simulink model "Simplus_Dual_Automated"  (R2022b)
settings: Solver=ode3  StartTime=0.0  StopTime=35  FixedStep=Ts  RelTol=1e-3  EnableMultiTasking=on
InitFcn:
  | Ts = 100e-6;
model workspace (MAT data in the model file):
  Fbase = 50
  Filter_Ind = 0.00435
  Shunt_C = 2.2e-06
  Test_Interval = 5
  Ts = 0.0001
  VDCref = 48
undefined symbols (not defined in the file): DiscIntNeverNeededParam
libraries: rtpi x45, spsabctodq0Lib x4, spsdq0toabcLib x2, simulink x1
(part 2 of 2)

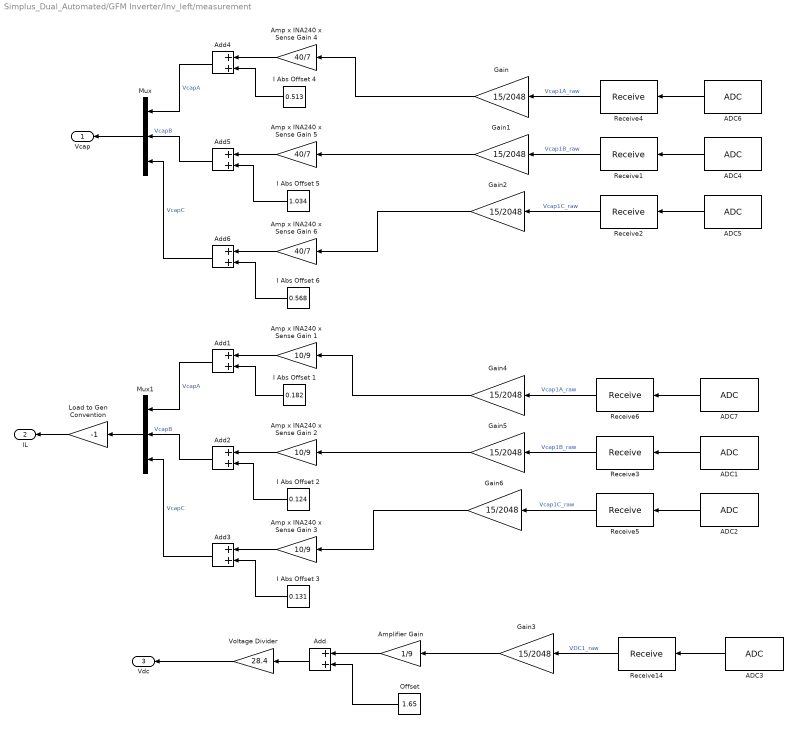
== system Simplus_Dual_Automated/GFM Inverter/Inv_left/measurement ==
  ADC1 : rtpi/ADC  finger_print=115482637925  blk_num=8  adcx=D  prior=2  pin=D2  trigger=PWM4A  data_type=int16  gain=1  rsrc=100  offset=AC  protect=Enabled  max=1500  min=-1500
      settings: SourceProductName=Simplus Real-Time
  ADC2 : rtpi/ADC  finger_print=115482637925  blk_num=9  adcx=D  prior=3  pin=D3  trigger=PWM4A  data_type=int16  gain=1  rsrc=100  offset=AC  protect=Enabled  max=1500  min=-1500
      settings: SourceProductName=Simplus Real-Time
  ADC3 : rtpi/ADC  finger_print=115482637925  blk_num=10  adcx=D  prior=4  pin=D4  trigger=PWM4A  data_type=int16  gain=1  rsrc=100  offset=AC  protect=Enabled  max=1500  min=-2048
      settings: SourceProductName=Simplus Real-Time
  ADC4 : rtpi/ADC  finger_print=115482637925  blk_num=11  adcx=C  prior=2  pin=C2  trigger=PWM4A  data_type=int16  gain=1  rsrc=100  offset=AC  protect=Enabled  max=1500  min=-1500
      settings: SourceProductName=Simplus Real-Time
  ADC5 : rtpi/ADC  finger_print=115482637925  blk_num=12  adcx=C  prior=3  pin=C3  trigger=PWM4A  data_type=int16  gain=1  rsrc=100  offset=AC  protect=Enabled  max=1500  min=-1500
      settings: SourceProductName=Simplus Real-Time
  ADC6 : rtpi/ADC  finger_print=115482637925  blk_num=13  adcx=C  prior=1  pin=C1  trigger=PWM4A  data_type=int16  gain=1  rsrc=100  offset=AC  protect=Enabled  max=1500  min=-1500
      settings: SourceProductName=Simplus Real-Time
  ADC7 : rtpi/ADC  finger_print=115482637925  blk_num=14  adcx=D  prior=1  pin=D1  trigger=PWM4A  data_type=int16  gain=1  rsrc=100  offset=AC  protect=Enabled  max=1500  min=-1500
      settings: SourceProductName=Simplus Real-Time
  Add{,1..6} (7 alike) : Sum
  Amp x INA240 x Sense Gain 1 : Gain  Gain=10/9
  Amp x INA240 x Sense Gain 2 : Gain  Gain=10/9
  Amp x INA240 x Sense Gain 3 : Gain  Gain=10/9
  Amp x INA240 x Sense Gain 4 : Gain  Gain=40/7
  Amp x INA240 x Sense Gain 5 : Gain  Gain=40/7
  Amp x INA240 x Sense Gain 6 : Gain  Gain=40/7
  Amplifier Gain : Gain  Gain=1/9
  Gain{,1..6} (7 alike) : Gain  Gain=15/2048
  I Abs Offset 1 : Constant  Value=0.182
  I Abs Offset 2 : Constant  Value=0.124
  I Abs Offset 3 : Constant  Value=0.131
  I Abs Offset 4 : Constant  Value=0.513
  I Abs Offset 5 : Constant  Value=1.034
  I Abs Offset 6 : Constant  Value=0.568
  Load to Gen Convention : Gain  Gain=-1
  Mux : Mux  Inputs=3
  Mux1 : Mux  Inputs=3
  Offset : Constant  Value=1.65
  Receive1 : rtpi/Receive  Priority=12  finger_print=115482637925  blk_num=8  data_type=2
      settings: SourceProductName=Simplus Real-Time
  Receive14 : rtpi/Receive  Priority=12  finger_print=115482637925  blk_num=9  data_type=2
      settings: SourceProductName=Simplus Real-Time
  Receive2 : rtpi/Receive  Priority=12  finger_print=115482637925  blk_num=10  data_type=2
      settings: SourceProductName=Simplus Real-Time
  Receive3 : rtpi/Receive  Priority=12  finger_print=115482637925  blk_num=11  data_type=2
      settings: SourceProductName=Simplus Real-Time
  Receive4 : rtpi/Receive  Priority=12  finger_print=115482637925  blk_num=12  data_type=2
      settings: SourceProductName=Simplus Real-Time
  Receive5 : rtpi/Receive  Priority=12  finger_print=115482637925  blk_num=13  data_type=2
      settings: SourceProductName=Simplus Real-Time
  Receive6 : rtpi/Receive  Priority=12  finger_print=115482637925  blk_num=14  data_type=2
      settings: SourceProductName=Simplus Real-Time
  Voltage Divider : Gain  Gain=28.4
  Vcap : Outport
  IL : Outport  Port=2
  Vdc : Outport  Port=3
  wires:
  ADC6/1 -> Receive4/1
  Receive4/1 -> Gain/1  "Vcap1A_raw"
  Amp x INA240 x Sense Gain 6/1 -> Add6/1
  I Abs Offset 6/1 -> Add6/2
  I Abs Offset 4/1 -> Add4/2
  Amp x INA240 x Sense Gain 4/1 -> Add4/1
  ADC5/1 -> Receive2/1
  Amp x INA240 x Sense Gain 5/1 -> Add5/1
  Receive1/1 -> Gain1/1  "Vcap1B_raw"
  I Abs Offset 5/1 -> Add5/2
  Receive2/1 -> Gain2/1  "Vcap1C_raw"
  ADC4/1 -> Receive1/1
  Amp x INA240 x Sense Gain 3/1 -> Add3/1
  Amp x INA240 x Sense Gain 1/1 -> Add1/1
  I Abs Offset 1/1 -> Add1/2
  Amp x INA240 x Sense Gain 2/1 -> Add2/1
  I Abs Offset 2/1 -> Add2/2
  I Abs Offset 3/1 -> Add3/2
  Receive14/1 -> Gain3/1  "VDC1_raw"
  ADC3/1 -> Receive14/1
  Add/1 -> Voltage Divider/1
  Amplifier Gain/1 -> Add/1
  Offset/1 -> Add/2
  Voltage Divider/1 -> Vdc/1
  Gain/1 -> Amp x INA240 x Sense Gain 4/1
  Gain1/1 -> Amp x INA240 x Sense Gain 5/1
  Gain2/1 -> Amp x INA240 x Sense Gain 6/1
  Gain3/1 -> Amplifier Gain/1
  Add4/1 -> Mux/1  "VcapA"
  Add5/1 -> Mux/2  "VcapB"
  Add6/1 -> Mux/3  "VcapC"
  Mux/1 -> Vcap/1
  ADC7/1 -> Receive6/1
  Gain4/1 -> Amp x INA240 x Sense Gain 1/1
  Gain5/1 -> Amp x INA240 x Sense Gain 2/1
  ADC1/1 -> Receive3/1
  ADC2/1 -> Receive5/1
  Receive3/1 -> Gain5/1  "Vcap1B_raw"
  Receive5/1 -> Gain6/1  "Vcap1C_raw"
  Gain6/1 -> Amp x INA240 x Sense Gain 3/1
  Receive6/1 -> Gain4/1  "Vcap1A_raw"
  Add3/1 -> Mux1/3  "VcapC"
  Mux1/1 -> Load to Gen Convention/1
  Add1/1 -> Mux1/1  "VcapA"
  Add2/1 -> Mux1/2  "VcapB"
  Load to Gen Convention/1 -> IL/1

== system Simplus_Dual_Automated/GFM Inverter/Voltage Controller/PI ==
  e : Inport
  RST : Inport  Port=2
  Discrete-Time Integrator : DiscreteIntegrator  gainval=1  ExternalReset=either  SampleTime=Ts  LimitOutput=on  UpperSaturationLimit=V_IntSat  LowerSaturationLimit=-V_IntSat  ICPrevOutput=DiscIntNeverNeededParam  ICPrevScaledInput=DiscIntNeverNeededParam
  Ki : Gain  Gain=Vd_Integral  SaturateOnIntegerOverflow=on  OutDataTypeStr=Inherit: Same as input  ParamDataTypeStr=Inherit: Same as input
  Kp : Gain  Gain=Vd_Proportional  SaturateOnIntegerOverflow=on  OutDataTypeStr=Inherit: Same as input  ParamDataTypeStr=Inherit: Same as input
  Sum4 : Sum  SaturateOnIntegerOverflow=on
  Out : Outport
  tag scope: GFM_Vd_Int_Out=global, GFM_Vd_PI_Out=global
  wires:
  Ki/1 -> Discrete-Time Integrator/1
  Kp/1 -> Sum4/1
  e/1 -> Ki/1, Kp/1
  Discrete-Time Integrator/1 -> [GFM_Vd_Int_Out], Sum4/2
  Sum4/1 -> [GFM_Vd_PI_Out], Out/1
  RST/1 -> Discrete-Time Integrator/2

== system Simplus_Dual_Automated/GFM Inverter/Voltage Controller/PI1 ==
  e : Inport
  RST : Inport  Port=2
  Discrete-Time Integrator : DiscreteIntegrator  gainval=1  ExternalReset=either  SampleTime=Ts  LimitOutput=on  UpperSaturationLimit=V_IntSat  LowerSaturationLimit=-V_IntSat  ICPrevOutput=DiscIntNeverNeededParam  ICPrevScaledInput=DiscIntNeverNeededParam
  Ki : Gain  Gain=Vd_Integral  SaturateOnIntegerOverflow=on  OutDataTypeStr=Inherit: Same as input  ParamDataTypeStr=Inherit: Same as input
  Kp : Gain  Gain=Vd_Proportional  SaturateOnIntegerOverflow=on  OutDataTypeStr=Inherit: Same as input  ParamDataTypeStr=Inherit: Same as input
  Sum4 : Sum  SaturateOnIntegerOverflow=on
  Out : Outport
  tag scope: GFM_Vq_Int_Out=global, GFM_Vq_PI_Out=global
  wires:
  Ki/1 -> Discrete-Time Integrator/1
  Kp/1 -> Sum4/1
  e/1 -> Ki/1, Kp/1
  RST/1 -> Discrete-Time Integrator/2
  Discrete-Time Integrator/1 -> [GFM_Vq_Int_Out], Sum4/2
  Sum4/1 -> [GFM_Vq_PI_Out], Out/1
